simulink model "LQI_Tentativa_Simulink"  (R2022a)
settings: Solver=VariableStepAuto  StartTime=0.0  StopTime=10  RelTol=1e-3
undefined symbols (not defined in the file): A, B, C, Kc_t, Ke_tbarra, Kf, Kf_t, Ki_t
settings Model: Creator=gabri  LastModifiedBy=gabri

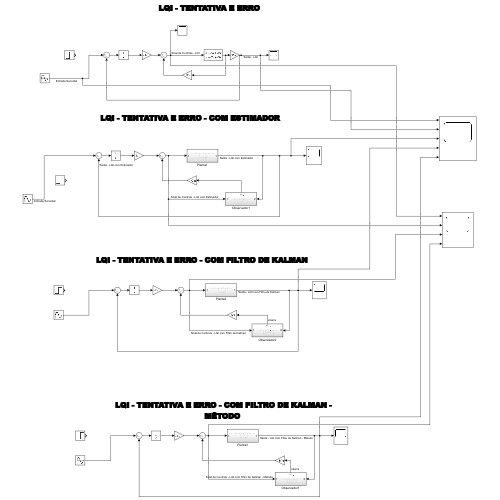
[thumbnail: Simulink's stored preview of the top-level diagram]
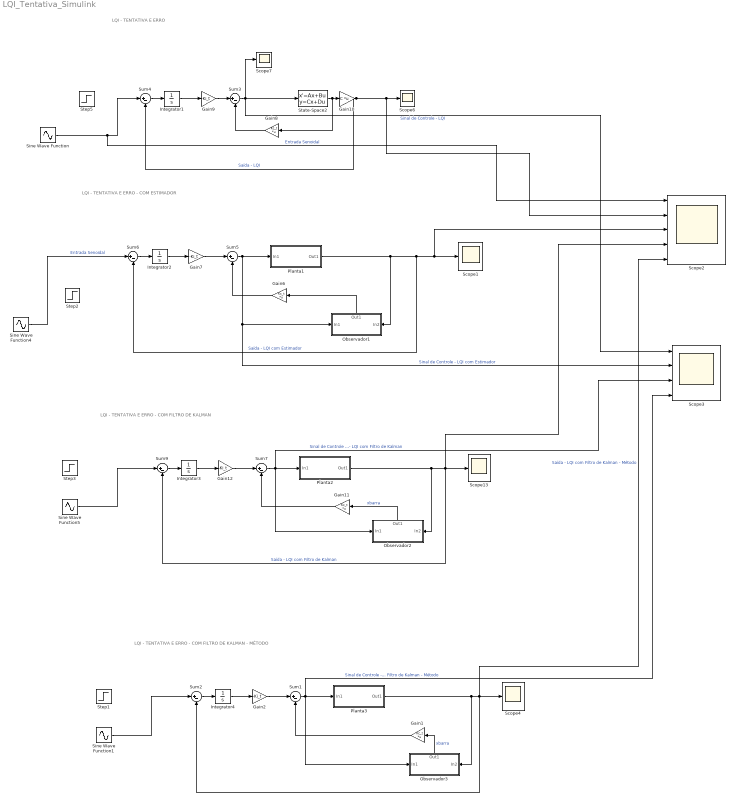
== system LQI_Tentativa_Simulink ==
  note: LQI - TENTATIVA E ERRO
  note: LQI - TENTATIVA E ERRO - COM ESTIMADOR
  note: LQI - TENTATIVA E ERRO - COM FILTRO DE KALMAN
  note: LQI - TENTATIVA E ERRO - COM FILTRO DE KALMAN - MÉTODO
  Gain{1,6,8,11} (4 alike) : Gain  Gain=Kc_t  Multiplication=Matrix(K*u)
  Gain10 : Gain  Gain=C  Multiplication=Matrix(K*u)
  Gain{2,7,9,12} (4 alike) : Gain  Gain=-Ki_t
  Integrator{1..4} (4 alike) : Integrator
  Observador1 : Subsystem
      settings: PortSchema="{\"entries\":[{\"content\":{\"sides\":[{\"content\":{\"connectorIds\":[\"In1\"]},\"type\":\"ConnectorPlacement.EquallySpacedRectSide\",\"uuid\":\"a39a08db-6117-4f96-90c3-02f1f7ffb9ec\"},{\"content\":{\"connectorIds\":[\"In2\"],\"side\":\"RIGHT\"},\"type\":\"ConnectorPlacement.EquallySpacedRectSide\",\"uuid\":\"e0a0a54b-1f6f-4425-9f49-01d22204810c\"},{\"content\":{\"connectorIds\":[\"Out1\"],\"side\":\"TOP\"},\"type\":\"ConnectorPlacement.EquallySpacedRectSide\",\"uuid\":\"f9c2d93e-7541-4a9e-b077-600f0b58f20b\"},{\"content\":{\"connectorIds\":[],\"side\":\"BOTTOM\"},\"type\":\"ConnectorPlacement.EquallySpacedRectSide\",\"uuid\":\"2e0212ac-38a2-465c-9330-e4bad70b5dfc\"}]},\"type\":\"ConnectorPlacement.EquallySpacedConnector\",\"uuid\":\"106c2d4c-b59c-4d15-84b9-899fdea4a460\"}],\"packageUris\":[\"http://schema.mathworks.com/mf0/Connector/R2020b\"],\"version\":\"1.0\"}"
  Observador2 : Subsystem
      settings: PortSchema="{\"entries\":[{\"content\":{\"sides\":[{\"content\":{\"connectorIds\":[\"In1\"]},\"type\":\"ConnectorPlacement.EquallySpacedRectSide\",\"uuid\":\"a39a08db-6117-4f96-90c3-02f1f7ffb9ec\"},{\"content\":{\"connectorIds\":[\"In2\"],\"side\":\"RIGHT\"},\"type\":\"ConnectorPlacement.EquallySpacedRectSide\",\"uuid\":\"e0a0a54b-1f6f-4425-9f49-01d22204810c\"},{\"content\":{\"connectorIds\":[\"Out1\"],\"side\":\"TOP\"},\"type\":\"ConnectorPlacement.EquallySpacedRectSide\",\"uuid\":\"f9c2d93e-7541-4a9e-b077-600f0b58f20b\"},{\"content\":{\"connectorIds\":[],\"side\":\"BOTTOM\"},\"type\":\"ConnectorPlacement.EquallySpacedRectSide\",\"uuid\":\"2e0212ac-38a2-465c-9330-e4bad70b5dfc\"}]},\"type\":\"ConnectorPlacement.EquallySpacedConnector\",\"uuid\":\"106c2d4c-b59c-4d15-84b9-899fdea4a460\"}],\"packageUris\":[\"http://schema.mathworks.com/mf0/Connector/R2020b\"],\"version\":\"1.0\"}"
  Observador3 : Subsystem
      settings: PortSchema="{\"entries\":[{\"content\":{\"sides\":[{\"content\":{\"connectorIds\":[\"In1\"]},\"type\":\"ConnectorPlacement.EquallySpacedRectSide\",\"uuid\":\"a39a08db-6117-4f96-90c3-02f1f7ffb9ec\"},{\"content\":{\"connectorIds\":[\"In2\"],\"side\":\"RIGHT\"},\"type\":\"ConnectorPlacement.EquallySpacedRectSide\",\"uuid\":\"e0a0a54b-1f6f-4425-9f49-01d22204810c\"},{\"content\":{\"connectorIds\":[\"Out1\"],\"side\":\"TOP\"},\"type\":\"ConnectorPlacement.EquallySpacedRectSide\",\"uuid\":\"f9c2d93e-7541-4a9e-b077-600f0b58f20b\"},{\"content\":{\"connectorIds\":[],\"side\":\"BOTTOM\"},\"type\":\"ConnectorPlacement.EquallySpacedRectSide\",\"uuid\":\"2e0212ac-38a2-465c-9330-e4bad70b5dfc\"}]},\"type\":\"ConnectorPlacement.EquallySpacedConnector\",\"uuid\":\"106c2d4c-b59c-4d15-84b9-899fdea4a460\"}],\"packageUris\":[\"http://schema.mathworks.com/mf0/Connector/R2020b\"],\"version\":\"1.0\"}"
  Planta1 : Subsystem
  Planta2 : Subsystem
  Planta3 : Subsystem
  Scope{1,4,6..7,13} (5 alike) : Scope
  Scope2 : Scope  NumInputPorts=5
  Scope3 : Scope  NumInputPorts=4
  Sine Wave Function{,1,4..5} (4 alike) : Sin  Amplitude=0.001  Frequency=pi  SampleTime=0
  State-Space2 : StateSpace  A=A  B=B  C=eye(3)  D=[0;0;0]  InitialCondition=0
  Step{1..3,5} (4 alike) : Step  Time=0  After=0.002  SampleTime=0
  Sum{1..7,9} (8 alike) : Sum  Inputs=|+-
  wires:
  Integrator1/1 -> Gain9/1
  Gain9/1 -> Sum3/1
  Gain10/1 -> Sum4/2, Scope2/2, Scope6/1  "Saída - LQI"
  Sum3/1 -> Scope3/1, State-Space2/1, Scope7/1  "Sinal de Controle - LQI"
  State-Space2/1 -> Gain8/1, Gain10/1
  Gain8/1 -> Sum3/2
  Sum4/1 -> Integrator1/1
  Gain7/1 -> Sum5/1
  Sum5/1 -> Planta1/1(In1), Scope3/2, Observador1/1(In1)  "Sinal de Controle - LQI com Estimador"
  Observador1/1(Out1) -> Gain6/1
  Integrator2/1 -> Gain7/1
  Gain6/1 -> Sum5/2
  Planta1/1(Out1) -> Observador1/2(In2), Scope2/3, Scope1/1, Sum6/2  "Saída - LQI com Estimador"
  Sum6/1 -> Integrator2/1
  Sum9/1 -> Integrator3/1
  Gain11/1 -> Sum7/2
  Gain12/1 -> Sum7/1
  Planta2/1(Out1) -> Observador2/2(In2), Scope2/4, Scope13/1, Sum9/2  "Saída - LQI com Filtro de Kalman"
  Sum7/1 -> Observador2/1(In1), Scope3/3, Planta2/1(In1)  "Sinal de Controle - LQI com Filtro de Kalman"
  Observador2/1(Out1) -> Gain11/1  "xbarra"
  Integrator3/1 -> Gain12/1
  Integrator4/1 -> Gain2/1
  Gain1/1 -> Sum1/2
  Sum1/1 -> Observador3/1(In1), Scope3/4, Planta3/1(In1)  "Sinal de Controle - LQI com Filtro de Kalman - Método"
  Sum2/1 -> Integrator4/1
  Observador3/1(Out1) -> Gain1/1  "xbarra"
  Gain2/1 -> Sum1/1
  Planta3/1(Out1) -> Observador3/2(In2), Scope2/5, Scope4/1, Sum2/2  "Saída - LQI com Filtro de Kalman - Método"
  Sine Wave Function/1 -> Scope2/1, Sum4/1  "Entrada Senoidal"
  Sine Wave Function5/1 -> Sum9/1
  Sine Wave Function1/1 -> Sum2/1
  Sine Wave Function4/1 -> Sum6/1  "Entrada Senoidal"

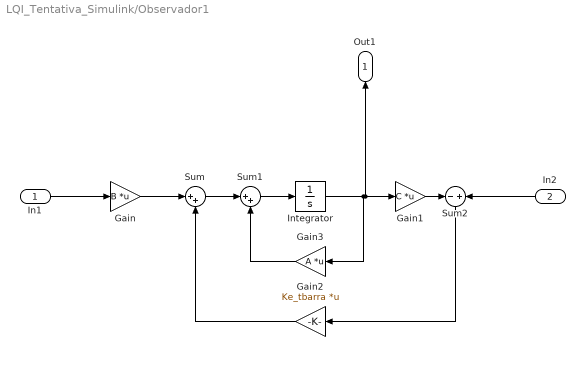
== system LQI_Tentativa_Simulink/Observador1 ==
  In1 : Inport
  In2 : Inport  Port=2
  Gain : Gain  Gain=B  Multiplication=Matrix(K*u)
  Gain1 : Gain  Gain=C  Multiplication=Matrix(K*u)
  Gain2 : Gain  Gain=Ke_tbarra  Multiplication=Matrix(K*u)
  Gain3 : Gain  Gain=A  Multiplication=Matrix(K*u)
  Integrator : Integrator
  Sum : Sum  Inputs=|++
  Sum1 : Sum  Inputs=|++
  Sum2 : Sum  Inputs=-|+
  Out1 : Outport
  wires:
  In1/1 -> Gain/1
  Gain/1 -> Sum/1
  Sum/1 -> Sum1/1
  Sum1/1 -> Integrator/1
  Integrator/1 -> Out1/1, Gain1/1, Gain3/1
  Gain1/1 -> Sum2/1
  In2/1 -> Sum2/2
  Sum2/1 -> Gain2/1
  Gain2/1 -> Sum/2
  Gain3/1 -> Sum1/2

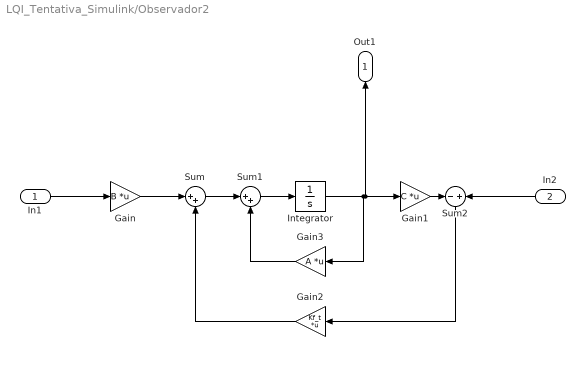
== system LQI_Tentativa_Simulink/Observador2 ==
  In1 : Inport
  In2 : Inport  Port=2
  Gain : Gain  Gain=B  Multiplication=Matrix(K*u)
  Gain1 : Gain  Gain=C  Multiplication=Matrix(K*u)
  Gain2 : Gain  Gain=Kf_t  Multiplication=Matrix(K*u)
  Gain3 : Gain  Gain=A  Multiplication=Matrix(K*u)
  Integrator : Integrator
  Sum : Sum  Inputs=|++
  Sum1 : Sum  Inputs=|++
  Sum2 : Sum  Inputs=-|+
  Out1 : Outport
  wires:
  In1/1 -> Gain/1
  Gain/1 -> Sum/1
  Sum/1 -> Sum1/1
  Sum1/1 -> Integrator/1
  Integrator/1 -> Out1/1, Gain1/1, Gain3/1
  Gain1/1 -> Sum2/1
  In2/1 -> Sum2/2
  Sum2/1 -> Gain2/1
  Gain2/1 -> Sum/2
  Gain3/1 -> Sum1/2

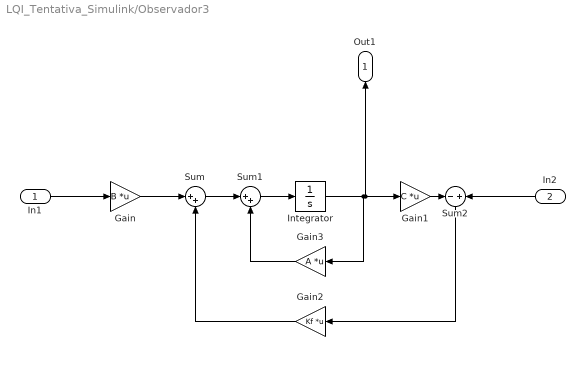
== system LQI_Tentativa_Simulink/Observador3 ==
  In1 : Inport
  In2 : Inport  Port=2
  Gain : Gain  Gain=B  Multiplication=Matrix(K*u)
  Gain1 : Gain  Gain=C  Multiplication=Matrix(K*u)
  Gain2 : Gain  Gain=Kf  Multiplication=Matrix(K*u)
  Gain3 : Gain  Gain=A  Multiplication=Matrix(K*u)
  Integrator : Integrator
  Sum : Sum  Inputs=|++
  Sum1 : Sum  Inputs=|++
  Sum2 : Sum  Inputs=-|+
  Out1 : Outport
  wires:
  In1/1 -> Gain/1
  Gain/1 -> Sum/1
  Sum/1 -> Sum1/1
  Sum1/1 -> Integrator/1
  Integrator/1 -> Out1/1, Gain1/1, Gain3/1
  Gain1/1 -> Sum2/1
  In2/1 -> Sum2/2
  Sum2/1 -> Gain2/1
  Gain2/1 -> Sum/2
  Gain3/1 -> Sum1/2

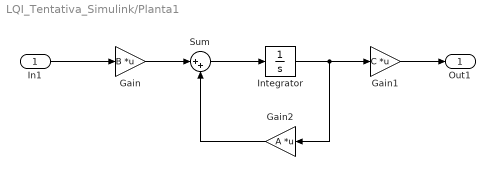
== system LQI_Tentativa_Simulink/Planta1 ==
  In1 : Inport
  Gain : Gain  Gain=B  Multiplication=Matrix(K*u)
  Gain1 : Gain  Gain=C  Multiplication=Matrix(K*u)
  Gain2 : Gain  Gain=A  Multiplication=Matrix(K*u)
  Integrator : Integrator
  Sum : Sum  Inputs=|++
  Out1 : Outport
  wires:
  In1/1 -> Gain/1
  Gain/1 -> Sum/1
  Sum/1 -> Integrator/1
  Integrator/1 -> Gain2/1, Gain1/1
  Gain1/1 -> Out1/1
  Gain2/1 -> Sum/2

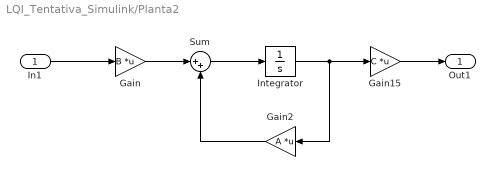
== system LQI_Tentativa_Simulink/Planta2 ==
  In1 : Inport
  Gain : Gain  Gain=B  Multiplication=Matrix(K*u)
  Gain15 : Gain  Gain=C  Multiplication=Matrix(K*u)
  Gain2 : Gain  Gain=A  Multiplication=Matrix(K*u)
  Integrator : Integrator
  Sum : Sum  Inputs=|++
  Out1 : Outport
  wires:
  In1/1 -> Gain/1
  Gain/1 -> Sum/1
  Sum/1 -> Integrator/1
  Integrator/1 -> Gain15/1, Gain2/1
  Gain2/1 -> Sum/2
  Gain15/1 -> Out1/1

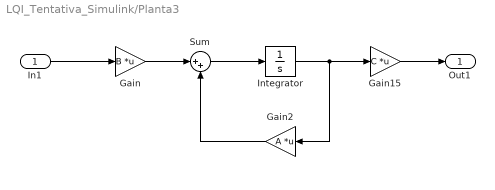
== system LQI_Tentativa_Simulink/Planta3 ==
  In1 : Inport
  Gain : Gain  Gain=B  Multiplication=Matrix(K*u)
  Gain15 : Gain  Gain=C  Multiplication=Matrix(K*u)
  Gain2 : Gain  Gain=A  Multiplication=Matrix(K*u)
  Integrator : Integrator
  Sum : Sum  Inputs=|++
  Out1 : Outport
  wires:
  In1/1 -> Gain/1
  Gain/1 -> Sum/1
  Sum/1 -> Integrator/1
  Integrator/1 -> Gain15/1, Gain2/1
  Gain2/1 -> Sum/2
  Gain15/1 -> Out1/1
